simulink model "simulink_travaux3"  (R2024a)
settings: Solver=VariableStepAuto  StartTime=0.0  StopTime=200  RelTol=1e-3
model workspace (MAT data in the model file):
  b_1 = Simulink.Parameter
  b_1.Complexity = 'real'
  b_1.Dimensions = [0 0]
  b_1.DataType = 'auto'
  b_2 = Simulink.Parameter
  b_2.Complexity = 'real'
  b_2.Dimensions = [0 0]
  b_2.DataType = 'auto'
  b_3 = Simulink.Parameter
  b_3.Complexity = 'real'
  b_3.Dimensions = [0 0]
  b_3.DataType = 'auto'
undefined symbols (not defined in the file): PID_DEN, PID_NUM
libraries: slpidlib x1
settings Model: Creator=OLPEL28  LastModifiedBy=OLPEL28

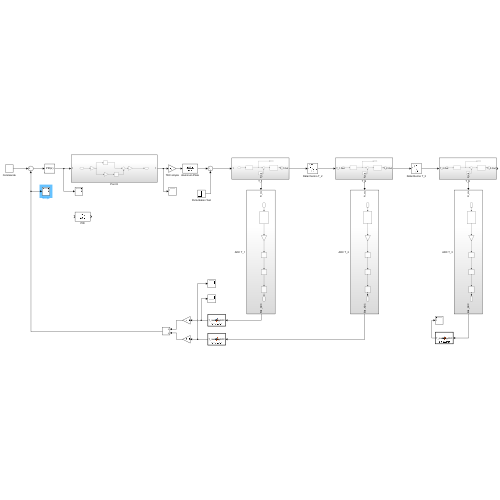
[thumbnail: Simulink's stored preview of the top-level diagram]
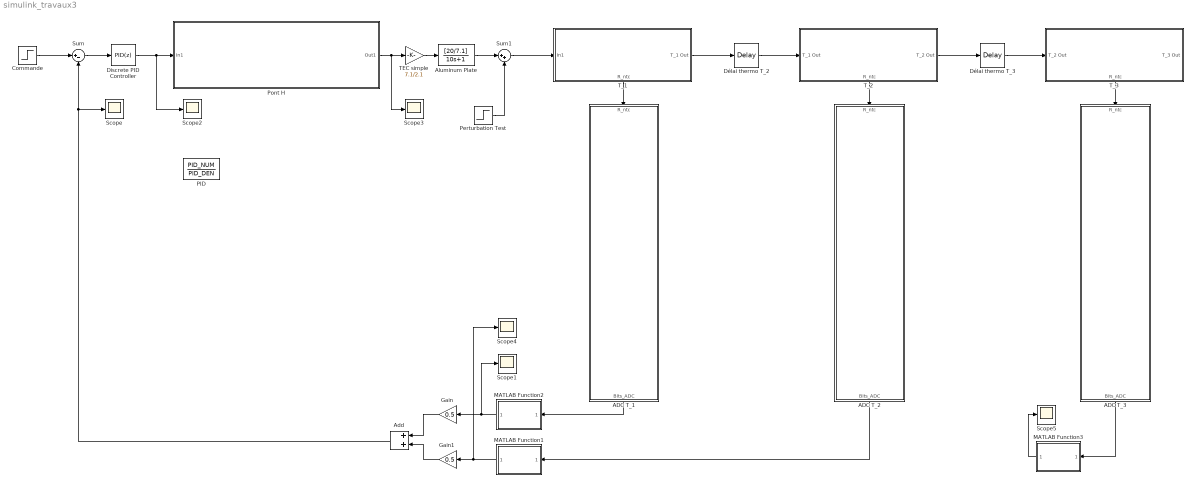
== system simulink_travaux3 ==
  ADC T_1 : Subsystem
  ADC T_2 : Subsystem
  ADC T_3 : Subsystem
  Add : Sum
  Aluminum Plate : TransferFcn  Numerator=[20/7.1]  Denominator=[10 1]
  Commande : Step  Time=0  Before=25  After=40  SampleTime=0
  Discrete PID Controller : slpidlib/PID Controller  Controller=PID  Form=Parallel  TimeDomain=Discrete-time  UseExternalTs=off  SampleTime=-1  IntegratorMethod=Forward Euler  FilterMethod=Forward Euler  ControllerParametersSource=internal  P=5  I=0.05  UseKiTs=off  D=1  UseExternalDerivativeSource=off  N=100  UseFilter=on  TunerSelectOption=Transfer Function Based (PID Tuner App)  InitialConditionSource=internal  InitialConditionForIntegrator=0  InitialConditionForFilter=0  DifferentiatorICPrevScaledInput=0  ExternalReset=none  TrackingMode=off  Kt=1  LimitOutput=off  SatLimitsSource=internal  UpperSaturationLimit=inf  LowerSaturationLimit=-inf  LinearizeAsGain=off  AntiWindupMode=none  Kb=1  LimitIntegrator=off  UpperIntegratorSaturationLimit=inf  LowerIntegratorSaturationLimit=-inf  POutMin=[]  POutMax=[]  IOutMin=[]  IOutMax=[]  DOutMin=[]  DOutMax=[]  NOutMin=[]  NOutMax=[]  SumOutMin=[]  SumOutMax=[]  SaturationOutMin=[]  SaturationOutMax=[]  PParamMin=[]  PParamMax=[]  IParamMin=[]  IParamMax=[]  DParamMin=[]  DParamMax=[]  NParamMin=[]  NParamMax=[]  KbParamMin=[]  KbParamMax=[]  KtParamMin=[]  KtParamMax=[]  KbOutMin=[]  KbOutMax=[]  KtOutMin=[]  KtOutMax=[]  IntegratorOutMin=[]  IntegratorOutMax=[]  FilterOutMin=[]  FilterOutMax=[]  SumI1OutMin=[]  SumI1OutMax=[]  SumI2OutMin=[]  SumI2OutMax=[]  SumI3OutMin=[]  SumI3OutMax=[]  SumI4OutMin=[]  SumI4OutMax=[]  SumDOutMin=[]  SumDOutMax=[]  DifferentiatorOutMin=[]  DifferentiatorOutMax=[]  FilterDiffOutCoefMin=[]  FilterDiffOutCoefMax=[]  ReciprocalOutMin=[]  ReciprocalOutMax=[]  SumDenOutMin=[]  SumDenOutMax=[]  SumNumOutMin=[]  SumNumOutMax=[]  DivideOutMin=[]  DivideOutMax=[]  UdiffTsProdOutMin=[]  UdiffTsProdOutMax=[]  NTsProdOutMin=[]  NTsProdOutMax=[]  UintegralTsProdOutMin=[]  UintegralTsProdOutMax=[]  UngainTsProdOutMin=[]  UngainTsProdOutMax=[]  ClampingZeroOutDataTypeStr=Inherit: Inherit via back propagation  ClampingZeroOutMin=[]  ClampingZeroOutMax=[]  FilterDenConstantOutDataTypeStr=Inherit: Inherit via back propagation  FilterDenConstantOutMin=[]  FilterDenConstantOutMax=[]  PCopyOutDataTypeStr=Inherit: Inherit via back propagation  PCopyOutMin=[]  PCopyOutMax=[]  NCopyOutDataTypeStr=Inherit: Inherit via back propagation  NCopyOutMin=[]  NCopyOutMax=[]  IntegratorContinuousStateAttributes=''  IntegratorStateMustResolveToSignalObject=off  IntegratorRTWStateStorageClass=Auto  FilterContinuousStateAttributes=''  FilterStateMustResolveToSignalObject=off  FilterRTWStateStorageClass=Auto  ParallelPVariant=InternalParameters  IdealPVariant=Disabled  IVariant=InternalParameters  DVariant=InternalParameters  IntegratorVariant=Discrete  SatVariant=Disabled  AWVariant=Passthrough  PCopyVariant=Disabled  TRVariant=Disabled  FdbkBlocksVariant=Forward  IdealPFdbkVariant=Disabled  SatFdbkVariant=Disabled  DerivativeFilterVariant=ForwardEulerFilter  NVariant=InternalParameters  NCopyVariant=Disabled  FilterICVariant=InternalICsFilter  IntegratorICVariant=InternalICs  ExternalResetVariant=Disabled  TRSumVariant=Passthrough  SumFdbkVariant=Disabled  SumVariant=Sum_PID  TsampFilterVariant=InternalTs  TsampNgainVariant=Passthrough  TsampIntegralVariant=Passthrough  ExternalSaturationOutDataTypeStr=Inherit: Same as second input  DerivativeSourceVariant=ErrorSignal
      settings: LibrarySourceBlock=simulink/Discrete/Discrete PID Controller
  Délai thermo T_2 : TransportDelay  DelayTime=7
  Délai thermo T_3 : TransportDelay  DelayTime=14
  Gain : Gain  Gain=0.5
  Gain1 : Gain  Gain=0.5
  MATLAB Function1 : MATLAB Function  TreatAsAtomicUnit=on
  MATLAB Function2 : MATLAB Function  TreatAsAtomicUnit=on
  MATLAB Function3 : MATLAB Function  TreatAsAtomicUnit=on
  PID : DiscreteTransferFcn  Numerator=PID_NUM  Denominator=PID_DEN
  Perturbation Test : Step  Time=0  After=0  SampleTime=0
  Pont H : Subsystem
  Scope{,1..5} (6 alike) : Scope
  Sum : Sum  Inputs=|+-
  Sum1 : Sum  Inputs=|++
  TEC simple : Gain  Gain=7.1/2.1
  T_1 : Subsystem
      settings: PortSchema="{\"entries\":[{\"content\":{\"sides\":[{\"content\":{\"connectorIds\":[\"In1\"]},\"type\":\"ConnectorPlacement.EquallySpacedRectSide\",\"uuid\":\"9022bc75-f2e1-4756-aed7-8214847faad0\"},{\"content\":{\"connectorIds\":[\"Out1\"],\"side\":\"RIGHT\"},\"type\":\"ConnectorPlacement.EquallySpacedRectSide\",\"uuid\":\"45d13b33-3548-4a7f-87ab-0833dbd02947\"},{\"content\":{\"side\":\"TOP\"},\"type\":\"ConnectorPlacement.EquallySpacedRectSide\",\"uuid\":\"2ac70de7-8112-4e76-971d-7a8ad18f41e6\"},{\"content\":{\"connectorIds\":[\"Out2\"],\"side\":\"BOTTOM\"},\"type\":\"ConnectorPlacement.EquallySpacedRectSide\",\"uuid\":\"b5357281-fab3-48c6-95cd-e6d21d6821fb\"}]},\"type\":\"ConnectorPlacement.EquallySpacedConnector\",\"uuid\":\"d4320567-c391-43ce-9cfc-be50ddc4307f\"}],\"packageUris\":[\"http://schema.mathworks.com/mf0/Connector/R2020b\"],\"version\":\"1.0\"}"
  T_2 : Subsystem
      settings: PortSchema="{\"entries\":[{\"content\":{\"sides\":[{\"content\":{\"connectorIds\":[\"In1\"]},\"type\":\"ConnectorPlacement.EquallySpacedRectSide\",\"uuid\":\"9022bc75-f2e1-4756-aed7-8214847faad0\"},{\"content\":{\"connectorIds\":[\"Out1\"],\"side\":\"RIGHT\"},\"type\":\"ConnectorPlacement.EquallySpacedRectSide\",\"uuid\":\"45d13b33-3548-4a7f-87ab-0833dbd02947\"},{\"content\":{\"side\":\"TOP\"},\"type\":\"ConnectorPlacement.EquallySpacedRectSide\",\"uuid\":\"2ac70de7-8112-4e76-971d-7a8ad18f41e6\"},{\"content\":{\"connectorIds\":[\"Out2\"],\"side\":\"BOTTOM\"},\"type\":\"ConnectorPlacement.EquallySpacedRectSide\",\"uuid\":\"b5357281-fab3-48c6-95cd-e6d21d6821fb\"}]},\"type\":\"ConnectorPlacement.EquallySpacedConnector\",\"uuid\":\"d4320567-c391-43ce-9cfc-be50ddc4307f\"}],\"packageUris\":[\"http://schema.mathworks.com/mf0/Connector/R2020b\"],\"version\":\"1.0\"}"
  T_3 : Subsystem
      settings: PortSchema="{\"entries\":[{\"content\":{\"sides\":[{\"content\":{\"connectorIds\":[\"In1\"]},\"type\":\"ConnectorPlacement.EquallySpacedRectSide\",\"uuid\":\"9022bc75-f2e1-4756-aed7-8214847faad0\"},{\"content\":{\"connectorIds\":[\"Out1\"],\"side\":\"RIGHT\"},\"type\":\"ConnectorPlacement.EquallySpacedRectSide\",\"uuid\":\"45d13b33-3548-4a7f-87ab-0833dbd02947\"},{\"content\":{\"side\":\"TOP\"},\"type\":\"ConnectorPlacement.EquallySpacedRectSide\",\"uuid\":\"2ac70de7-8112-4e76-971d-7a8ad18f41e6\"},{\"content\":{\"connectorIds\":[\"Out2\"],\"side\":\"BOTTOM\"},\"type\":\"ConnectorPlacement.EquallySpacedRectSide\",\"uuid\":\"b5357281-fab3-48c6-95cd-e6d21d6821fb\"}]},\"type\":\"ConnectorPlacement.EquallySpacedConnector\",\"uuid\":\"d4320567-c391-43ce-9cfc-be50ddc4307f\"}],\"packageUris\":[\"http://schema.mathworks.com/mf0/Connector/R2020b\"],\"version\":\"1.0\"}"
  wires:
  Commande/1 -> Sum/1
  Perturbation Test/1 -> Sum1/2
  TEC simple/1 -> Aluminum Plate/1
  Pont H/1(Out1) -> Scope3/1, TEC simple/1
  Sum1/1 -> T_1/1(In1)
  T_1/2(R_ntc) -> ADC T_1/1(R_ntc)
  T_2/2(R_ntc) -> ADC T_2/1(R_ntc)
  ADC T_1/1(Bits_ADC) -> MATLAB Function2/1(Bits_ADC)
  ADC T_2/1(Bits_ADC) -> MATLAB Function1/1(Bits_ADC)
  T_1/1(T_1 Out) -> Délai thermo T_2/1
  Délai thermo T_2/1 -> T_2/1(T_1 Out)
  Aluminum Plate/1 -> Sum1/1
  MATLAB Function2/1(T_mesuree) -> Scope1/1, Gain/1
  MATLAB Function1/1(T_mesuree) -> Scope4/1, Gain1/1
  Gain1/1 -> Add/2
  Gain/1 -> Add/1
  Add/1 -> Scope/1, Sum/2
  Délai thermo T_3/1 -> T_3/1(T_2 Out)
  T_3/2(R_ntc) -> ADC T_3/1(R_ntc)
  T_2/1(T_2 Out) -> Délai thermo T_3/1
  ADC T_3/1(Bits_ADC) -> MATLAB Function3/1(Bits_ADC)
  MATLAB Function3/1(T_mesuree) -> Scope5/1
  Sum/1 -> Discrete PID Controller/1
  Discrete PID Controller/1 -> Scope2/1, Pont H/1(In1)

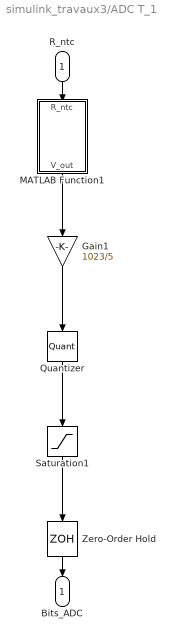
== system simulink_travaux3/ADC T_1 ==
  R_ntc : Inport
  Gain1 : Gain  Gain=1023/5
  MATLAB Function1 : MATLAB Function  TreatAsAtomicUnit=on
  Quantizer : Quantizer  QuantizationInterval=1
  Saturation1 : Saturate  UpperLimit=1023  LowerLimit=0
  Zero-Order Hold : ZeroOrderHold  SampleTime=0.01
  Bits_ADC : Outport
  wires:
  Quantizer/1 -> Saturation1/1
  Gain1/1 -> Quantizer/1
  Saturation1/1 -> Zero-Order Hold/1
  Zero-Order Hold/1 -> Bits_ADC/1
  R_ntc/1 -> MATLAB Function1/1(R_ntc)
  MATLAB Function1/1(V_out) -> Gain1/1

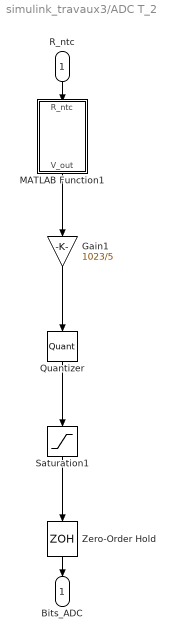
== system simulink_travaux3/ADC T_2 ==
  R_ntc : Inport
  Gain1 : Gain  Gain=1023/5
  MATLAB Function1 : MATLAB Function  TreatAsAtomicUnit=on
  Quantizer : Quantizer  QuantizationInterval=1
  Saturation1 : Saturate  UpperLimit=1023  LowerLimit=0
  Zero-Order Hold : ZeroOrderHold  SampleTime=0.01
  Bits_ADC : Outport
  wires:
  Quantizer/1 -> Saturation1/1
  Gain1/1 -> Quantizer/1
  Saturation1/1 -> Zero-Order Hold/1
  Zero-Order Hold/1 -> Bits_ADC/1
  R_ntc/1 -> MATLAB Function1/1(R_ntc)
  MATLAB Function1/1(V_out) -> Gain1/1

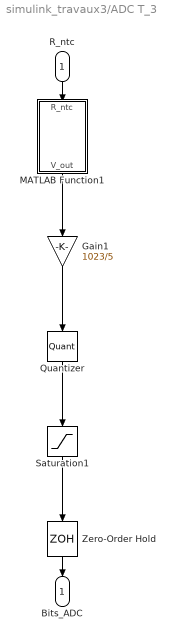
== system simulink_travaux3/ADC T_3 ==
  R_ntc : Inport
  Gain1 : Gain  Gain=1023/5
  MATLAB Function1 : MATLAB Function  TreatAsAtomicUnit=on
  Quantizer : Quantizer  QuantizationInterval=1
  Saturation1 : Saturate  UpperLimit=1023  LowerLimit=0
  Zero-Order Hold : ZeroOrderHold  SampleTime=0.01
  Bits_ADC : Outport
  wires:
  Quantizer/1 -> Saturation1/1
  Gain1/1 -> Quantizer/1
  Saturation1/1 -> Zero-Order Hold/1
  Zero-Order Hold/1 -> Bits_ADC/1
  R_ntc/1 -> MATLAB Function1/1(R_ntc)
  MATLAB Function1/1(V_out) -> Gain1/1

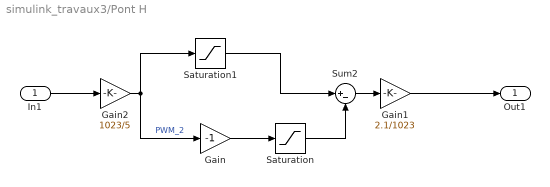
== system simulink_travaux3/Pont H ==
  In1 : Inport
  Gain : Gain  Gain=-1
  Gain1 : Gain  Gain=2.1/1023
  Gain2 : Gain  Gain=1023/5
  Saturation : Saturate  UpperLimit=1023  LowerLimit=0
  Saturation1 : Saturate  UpperLimit=1023  LowerLimit=0
  Sum2 : Sum  Inputs=|+-
  Out1 : Outport
  wires:
  Saturation1/1 -> Sum2/1
  Saturation/1 -> Sum2/2
  Sum2/1 -> Gain1/1
  Gain1/1 -> Out1/1
  Gain2/1 -> Saturation1/1, Gain/1  "PWM_2"
  Gain/1 -> Saturation/1
  In1/1 -> Gain2/1

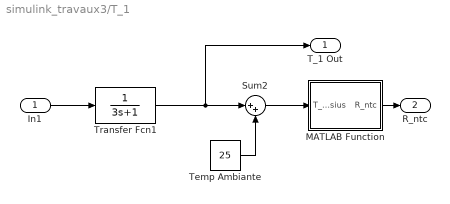
== system simulink_travaux3/T_1 ==
  In1 : Inport
  MATLAB Function : MATLAB Function  TreatAsAtomicUnit=on
  Sum2 : Sum  Inputs=|++
  Temp Ambiante : Constant  Value=25
  Transfer Fcn1 : TransferFcn  Denominator=[3 1]
  T_1 Out : Outport
  R_ntc : Outport  Port=2
  wires:
  Transfer Fcn1/1 -> Sum2/1, T_1 Out/1
  MATLAB Function/1(R_ntc) -> R_ntc/1
  In1/1 -> Transfer Fcn1/1
  Sum2/1 -> MATLAB Function/1(T_celsius)
  Temp Ambiante/1 -> Sum2/2

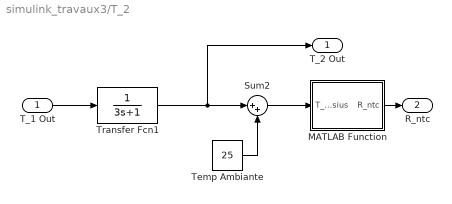
== system simulink_travaux3/T_2 ==
  T_1 Out : Inport
  MATLAB Function : MATLAB Function  TreatAsAtomicUnit=on
  Sum2 : Sum  Inputs=|++
  Temp Ambiante : Constant  Value=25
  Transfer Fcn1 : TransferFcn  Denominator=[3 1]
  T_2 Out : Outport
  R_ntc : Outport  Port=2
  wires:
  Transfer Fcn1/1 -> Sum2/1, T_2 Out/1
  MATLAB Function/1(R_ntc) -> R_ntc/1
  T_1 Out/1 -> Transfer Fcn1/1
  Temp Ambiante/1 -> Sum2/2
  Sum2/1 -> MATLAB Function/1(T_celsius)

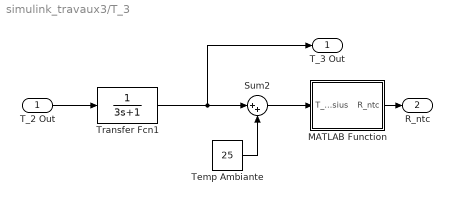
== system simulink_travaux3/T_3 ==
  T_2 Out : Inport
  MATLAB Function : MATLAB Function  TreatAsAtomicUnit=on
  Sum2 : Sum  Inputs=|++
  Temp Ambiante : Constant  Value=25
  Transfer Fcn1 : TransferFcn  Denominator=[3 1]
  T_3 Out : Outport
  R_ntc : Outport  Port=2
  wires:
  Transfer Fcn1/1 -> Sum2/1, T_3 Out/1
  MATLAB Function/1(R_ntc) -> R_ntc/1
  T_2 Out/1 -> Transfer Fcn1/1
  Temp Ambiante/1 -> Sum2/2
  Sum2/1 -> MATLAB Function/1(T_celsius)

== matlab function simulink_travaux3/T_1/MATLAB Function ==
  data: T_celsius input; R_ntc output
function R_ntc = temp2res(T_celsius)
    % Paramètres de la thermistance NTCALUG02A
    R25 = 10000;      % 10k Ohms à 25°C
    T25 = 298.15;     % 25°C en Kelvin
    Beta = 3984;      % Valeur B25/85 du tableau

    T_kelvin = T_celsius + 273.15;
    
    % Équation simplifiée de Steinhart-Hart (Parameter B)
    R_ntc = R25 * exp(Beta * (1/T_kelvin - 1/T25));
end

== matlab function simulink_travaux3/MATLAB Function2 ==
  data: Bits_ADC input; T_mesuree output
function T_mesuree = bits2temp(Bits_ADC)
    % Inverse exact de la chaîne précédente
    V_source = 5;
    R_fixe = 10000;
    R25 = 10000;
    T25 = 298.15;
    Beta = 3984;

    % 1. Bits en Voltage
    V_mes = (Bits_ADC * V_source) / 1023;
    
    % 2. Voltage en Résistance (Inverse du pont diviseur)
    % Attention à la division par zéro si V_mes est proche de V_source
    R_ntc = (V_mes * R_fixe) / (V_source - V_mes);
    
    % 3. Résistance en Température (Inverse Steinhart-Hart)
    T_kelvin = 1 / ( (1/Beta) * log(R_ntc/R25) + (1/T25) );
    
    T_mesuree = T_kelvin - 273.15;
end

== matlab function simulink_travaux3/T_2/MATLAB Function ==
  data: T_celsius input; R_ntc output
function R_ntc = temp2res(T_celsius)
    % Paramètres de la thermistance NTCALUG02A
    R25 = 10000;      % 10k Ohms à 25°C
    T25 = 298.15;     % 25°C en Kelvin
    Beta = 3984;      % Valeur B25/85 du tableau

    T_kelvin = T_celsius + 273.15;
    
    % Équation simplifiée de Steinhart-Hart (Parameter B)
    R_ntc = R25 * exp(Beta * (1/T_kelvin - 1/T25));
end

== matlab function simulink_travaux3/ADC T_2/MATLAB Function1 ==
  data: R_ntc input; V_out output
function V_out = res2volt(R_ntc)
    V_source = 5;     % Arduino fonctionne en 5V
    R_fixe = 10000;   % Résistance du pont diviseur (À VÉRIFIER sur ton PCB!)
    
    % Formule du diviseur de tension
    V_out = V_source * (R_ntc / (R_ntc + R_fixe));
end

== matlab function simulink_travaux3/MATLAB Function1 ==
  data: Bits_ADC input; T_mesuree output
function T_mesuree = bits2temp(Bits_ADC)
    % Inverse exact de la chaîne précédente
    V_source = 5;
    R_fixe = 10000;
    R25 = 10000;
    T25 = 298.15;
    Beta = 3984;

    % 1. Bits en Voltage
    V_mes = (Bits_ADC * V_source) / 1023;
    
    % 2. Voltage en Résistance (Inverse du pont diviseur)
    % Attention à la division par zéro si V_mes est proche de V_source
    R_ntc = (V_mes * R_fixe) / (V_source - V_mes);
    
    % 3. Résistance en Température (Inverse Steinhart-Hart)
    T_kelvin = 1 / ( (1/Beta) * log(R_ntc/R25) + (1/T25) );
    
    T_mesuree = T_kelvin - 273.15;
end

== matlab function simulink_travaux3/ADC T_3/MATLAB Function1 ==
  data: R_ntc input; V_out output
function V_out = res2volt(R_ntc)
    V_source = 5;     % Arduino fonctionne en 5V
    R_fixe = 10000;   % Résistance du pont diviseur (À VÉRIFIER sur ton PCB!)
    
    % Formule du diviseur de tension
    V_out = V_source * (R_ntc / (R_ntc + R_fixe));
end

== matlab function simulink_travaux3/T_3/MATLAB Function ==
  data: T_celsius input; R_ntc output
function R_ntc = temp2res(T_celsius)
    % Paramètres de la thermistance NTCALUG02A
    R25 = 10000;      % 10k Ohms à 25°C
    T25 = 298.15;     % 25°C en Kelvin
    Beta = 3984;      % Valeur B25/85 du tableau

    T_kelvin = T_celsius + 273.15;
    
    % Équation simplifiée de Steinhart-Hart (Parameter B)
    R_ntc = R25 * exp(Beta * (1/T_kelvin - 1/T25));
end

== matlab function simulink_travaux3/MATLAB Function3 ==
  data: Bits_ADC input; T_mesuree output
function T_mesuree = bits2temp(Bits_ADC)
    % Inverse exact de la chaîne précédente
    V_source = 5;
    R_fixe = 10000;
    R25 = 10000;
    T25 = 298.15;
    Beta = 3984;

    % 1. Bits en Voltage
    V_mes = (Bits_ADC * V_source) / 1023;
    
    % 2. Voltage en Résistance (Inverse du pont diviseur)
    % Attention à la division par zéro si V_mes est proche de V_source
    R_ntc = (V_mes * R_fixe) / (V_source - V_mes);
    
    % 3. Résistance en Température (Inverse Steinhart-Hart)
    T_kelvin = 1 / ( (1/Beta) * log(R_ntc/R25) + (1/T25) );
    
    T_mesuree = T_kelvin - 273.15;
end

== matlab function simulink_travaux3/ADC T_1/MATLAB Function1 ==
  data: R_ntc input; V_out output
function V_out = res2volt(R_ntc)
    V_source = 5;     % Arduino fonctionne en 5V
    R_fixe = 10000;   % Résistance du pont diviseur (À VÉRIFIER sur ton PCB!)
    
    % Formule du diviseur de tension
    V_out = V_source * (R_ntc / (R_ntc + R_fixe));
end
